simulink model "Assembly"  (R2022b)
settings: Solver=FixedStepAuto  StartTime=0.0  StopTime=20  FixedStep=0.001  RelTol=1e-3
model workspace: external: MATLAB File D:\Bw Jiang\Documents\FCS\DuctedFanUAV\Assembly_DataFile.m (data not in the file)
undefined symbols (not defined in the file or in its folder): DiscIntNeverNeededParam, smiData, X, Y, Z
libraries: sm_lib x26, nesl_utility x21, slpidlib x18, simulink_extras x5, simulink x4, shared6dof x2
(part 1 of 4)
settings Model: PacingRate=0.250000  Creator=Bw Jiang  LastModifiedBy=Bw Jiang
settings DebuggingCC: UnconnectedInputMsg=warning  UnconnectedOutputMsg=warning  UnconnectedLineMsg=warning
settings ModelReferenceCC: EnableRefExpFcnMdlSchedulingChecks=on
settings RTWCC: DLArmComputeVersion=19.05

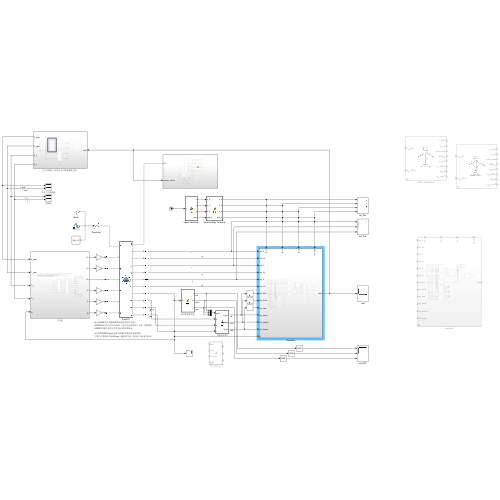
[thumbnail: Simulink's stored preview of the top-level diagram]
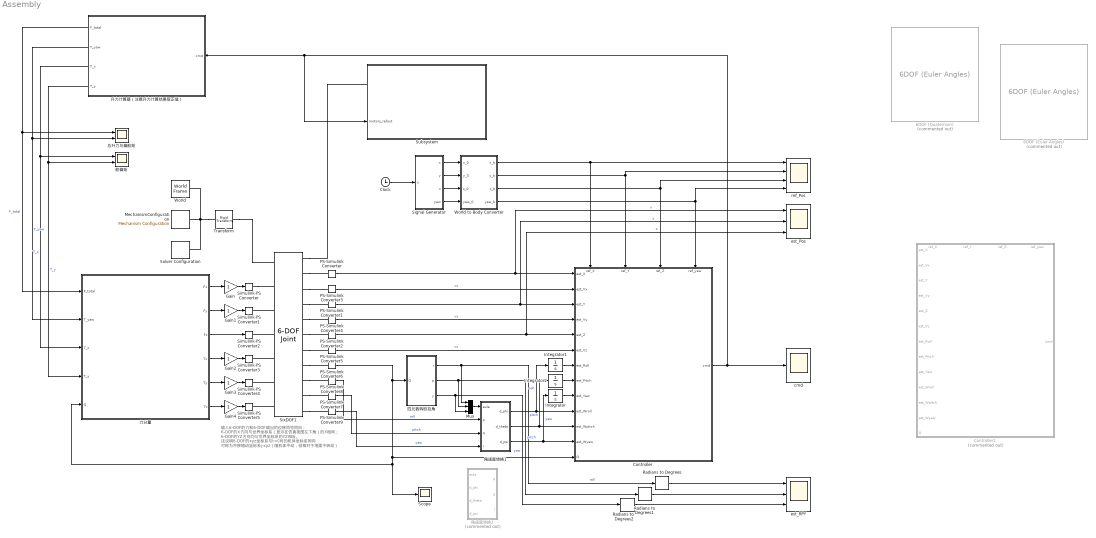
== system Assembly ==
  note: 输入6-DOF的力和6-DOF输出的位移同号同向；
      | 6-DOF的X方向与世界坐标系（显示在仿真视图左下角）的X相同；
      | 6-DOF的YZ方向均与世界坐标系的YZ相反。
      |
      | 这说明6-DOF的xyz坐标系与t=0时的机体坐标系同向
      | 可称为平移随动坐标系j-xyz（随机体平动，但相对于地面不转动）
  6DOF (Euler Angles) : shared6dof/6DOF (Euler Angles)  Commented=on  units=Metric (MKS)  mtype=Fixed  rep=Euler Angles  xme_0=[0 0 0]  Vm_0=[0 0 0]  eul_0=[0 0 0]  pm_0=[0 0 0]  mass_0=1.0  mass_e=0.5  mass_f=2.0  inertia=eye(3)  inertia_e=eye(3)  inertia_f=2*eye(3)  k_quat=1.0  vre_flag=on  abi_flag=off  aMode=0  xme_statename=''  Vm_statename=''  eul_statename=''  quat_statename=''  pm_statename=''  mass_statename=''
  6DOF (Quaternion) : shared6dof/6DOF (Euler Angles)  Commented=on  units=Metric (MKS)  mtype=Fixed  rep=Quaternion  xme_0=[0 0 0]  Vm_0=[0 0 0]  eul_0=[0 0 0]  pm_0=[0 0 0]  mass_0=1.0  mass_e=0.5  mass_f=2.0  inertia=eye(3)  inertia_e=eye(3)  inertia_f=2*eye(3)  k_quat=1.0  vre_flag=on  abi_flag=off  aMode=0  xme_statename=''  Vm_statename=''  eul_statename=''  quat_statename=''  pm_statename=''  mass_statename=''
  Clock : Clock
  Controller : Subsystem
      settings: PortSchema="{\"entries\":[{\"content\":{\"sides\":[{\"content\":{\"connectorIds\":[\"In1\",\"In2\",\"In3\",\"In4\",\"In5\",\"In6\",\"In7\",\"In8\",\"In9\",\"In10\",\"In11\",\"In12\",\"In13\"]},\"type\":\"ConnectorPlacement.EquallySpacedRectSide\",\"uuid\":\"809a58d1-8f24-4346-a9a1-bdf3f40071a9\"},{\"content\":{\"connectorIds\":[\"Out1\"],\"side\":\"RIGHT\"},\"type\":\"ConnectorPlacement.EquallySpacedRectSide\",\"uuid\":\"e36db7a5-8644-49ff-9b48-8e381d81be19\"},{\"content\":{\"connectorIds\":[\"In14\",\"In15\",\"In16\",\"In17\"],\"side\":\"TOP\"},\"type\":\"ConnectorPlacement.EquallySpacedRectSide\",\"uuid\":\"d8c211b6-7652-4be5-9d63-16c6c31a5cb3\"}]},\"type\":\"ConnectorPlacement.EquallySpacedConnector\",\"uuid\":\"28a38415-8484-4982-8141-ea2d794bbc37\"}],\"packageUris\":[\"http://schema.mathworks.com/mf0/Connector/R2020b\"],\"version\":\"1.0\"}"
  Controller1 : Subsystem  Commented=on
      settings: PortSchema="{\"entries\":[{\"content\":{\"sides\":[{\"content\":{\"connectorIds\":[\"In1\",\"In2\",\"In3\",\"In4\",\"In5\",\"In6\",\"In7\",\"In8\",\"In9\",\"In10\",\"In11\",\"In12\",\"In13\"]},\"type\":\"ConnectorPlacement.EquallySpacedRectSide\",\"uuid\":\"809a58d1-8f24-4346-a9a1-bdf3f40071a9\"},{\"content\":{\"connectorIds\":[\"Out1\"],\"side\":\"RIGHT\"},\"type\":\"ConnectorPlacement.EquallySpacedRectSide\",\"uuid\":\"e36db7a5-8644-49ff-9b48-8e381d81be19\"},{\"content\":{\"connectorIds\":[\"In14\",\"In15\",\"In16\",\"In17\"],\"side\":\"TOP\"},\"type\":\"ConnectorPlacement.EquallySpacedRectSide\",\"uuid\":\"d8c211b6-7652-4be5-9d63-16c6c31a5cb3\"}]},\"type\":\"ConnectorPlacement.EquallySpacedConnector\",\"uuid\":\"28a38415-8484-4982-8141-ea2d794bbc37\"}],\"packageUris\":[\"http://schema.mathworks.com/mf0/Connector/R2020b\"],\"version\":\"1.0\"}"
  Gain{,1..4} (5 alike) : Gain
  Integrator : Integrator
  Integrator1 : Integrator
  Integrator2 : Integrator
  MechanismConfiguration : sm_lib/Utilities/Mechanism Configuration  UniformGravity=Constant  GravityVector=[0 0 -9.81]  GravityUnits=m/s^2  LinearizationDelta=0.001  JointModeTransitionNonlinearIterations=2
  Mux : Mux  Inputs=3
  PS-Simulink Converter{,1..9} (10 alike) : nesl_utility/PS-Simulink Converter  PhysicalDomain=network_engine_domain  SubClassName=ps_output  LeftPortType=input  RightPortType=output  PseudoPeriodic=off  Frequencies=[]  VectorFormat=1-D array  Unit=inherit  AffineConversion=off
  Radians to Degrees : simulink_extras/Transformations/Radians to Degrees
  Radians to Degrees1 : simulink_extras/Transformations/Radians to Degrees
  Radians to Degrees2 : simulink_extras/Transformations/Radians to Degrees
  Scope : Scope
  Signal Generator : MATLAB Function  TreatAsAtomicUnit=on
  Simulink-PS Converter{,1..5} (6 alike) : nesl_utility/Simulink-PS Converter  PhysicalDomain=network_engine_domain  SubClassName=ps_input  LeftPortType=input  RightPortType=output  PseudoPeriodic=off  Frequencies=[]  NoiseDistribution=none  NoiseParameters=[]  Unit=1  AffineConversion=off  FilteringAndDerivatives=provide  SimscapeFilterOrder=1  InputFilterTimeConstant=0.001  UdotUserProvided=0
  SixDOF1 : sm_lib/Joints/6-DOF Joint  JointMode=Normal  SenseConstraintForce=off  SenseConstraintForceX=off  SenseConstraintForceY=off  SenseConstraintForceZ=off  SenseConstraintTorque=off  SenseConstraintTorqueX=off  SenseConstraintTorqueY=off  SenseConstraintTorqueZ=off  SenseTotalForce=off  SenseTotalForceX=off  SenseTotalForceY=off  SenseTotalForceZ=off  SenseTotalTorque=off  SenseTotalTorqueX=off  SenseTotalTorqueY=off  SenseTotalTorqueZ=off  CompositeWrenchDir=FollowerOnBase  CompositeWrenchFrame=BaseFrame  PxEquilibriumPosition=0  PxEquilibriumPositionUnits=m  PxSpringStiffness=0  PxSpringStiffnessUnits=N/m  PxDampingCoefficient=0  PxDampingCoefficientUnits=N/(m/s)  PxTorqueActuationMode=InputTorque  PxMotionActuationMode=ComputedMotion  PxSensePosition=on  PxSenseVelocity=on  PxSenseAcceleration=off  PxSenseTorqueForce=off  PxSenseLowerLimitTorqueForce=off  PxSenseUpperLimitTorqueForce=off  PxLowerLimitSpecify=off  PxLowerLimitBound=-1  PxLowerLimitBoundUnits=m  PxLowerLimitStiffness=1e6  PxLowerLimitStiffnessUnits=N/m  PxLowerLimitDamping=1e3  PxLowerLimitDampingUnits=N/(m/s)  PxLowerLimitTransitionRegionWidth=1e-4  PxLowerLimitTransitionRegionWidthUnits=m  PxUpperLimitSpecify=off  PxUpperLimitBound=1  PxUpperLimitBoundUnits=m  PxUpperLimitStiffness=1e6  PxUpperLimitStiffnessUnits=N/m  PxUpperLimitDamping=1e3  PxUpperLimitDampingUnits=N/(m/s)  PxUpperLimitTransitionRegionWidth=1e-4  PxUpperLimitTransitionRegionWidthUnits=m  PxPositionTargetSpecify=off  PxPositionTargetPriority=High  PxPositionTargetValue=0  PxPositionTargetValueUnits=m  PxVelocityTargetSpecify=off  PxVelocityTargetPriority=High  PxVelocityTargetValue=0  PxVelocityTargetValueUnits=m/s  PyEquilibriumPosition=0  PyEquilibriumPositionUnits=m  PySpringStiffness=0  PySpringStiffnessUnits=N/m  PyDampingCoefficient=0  PyDampingCoefficientUnits=N/(m/s)  PyTorqueActuationMode=InputTorque  PyMotionActuationMode=ComputedMotion  PySensePosition=on  PySenseVelocity=on  PySenseAcceleration=off  PySenseTorqueForce=off  PySenseLowerLimitTorqueForce=off  PySenseUpperLimitTorqueForce=off  PyLowerLimitSpecify=off  PyLowerLimitBound=-1  PyLowerLimitBoundUnits=m  PyLowerLimitStiffness=1e6  PyLowerLimitStiffnessUnits=N/m  PyLowerLimitDamping=1e3  PyLowerLimitDampingUnits=N/(m/s)  PyLowerLimitTransitionRegionWidth=1e-4  PyLowerLimitTransitionRegionWidthUnits=m  PyUpperLimitSpecify=off  PyUpperLimitBound=1  PyUpperLimitBoundUnits=m  PyUpperLimitStiffness=1e6  PyUpperLimitStiffnessUnits=N/m  PyUpperLimitDamping=1e3  PyUpperLimitDampingUnits=N/(m/s)  PyUpperLimitTransitionRegionWidth=1e-4  PyUpperLimitTransitionRegionWidthUnits=m  PyPositionTargetSpecify=off  PyPositionTargetPriority=High  PyPositionTargetValue=0  PyPositionTargetValueUnits=m  PyVelocityTargetSpecify=off  PyVelocityTargetPriority=High  PyVelocityTargetValue=0  PyVelocityTargetValueUnits=m/s  PzEquilibriumPosition=0  PzEquilibriumPositionUnits=m  PzSpringStiffness=0  PzSpringStiffnessUnits=N/m  PzDampingCoefficient=0  PzDampingCoefficientUnits=N/(m/s)  PzTorqueActuationMode=InputTorque  PzMotionActuationMode=ComputedMotion  PzSensePosition=on  PzSenseVelocity=on  PzSenseAcceleration=off  PzSenseTorqueForce=off  PzSenseLowerLimitTorqueForce=off  PzSenseUpperLimitTorqueForce=off  PzLowerLimitSpecify=off  PzLowerLimitBound=-1  PzLowerLimitBoundUnits=m  PzLowerLimitStiffness=1e6  PzLowerLimitStiffnessUnits=N/m  PzLowerLimitDamping=1e3  PzLowerLimitDampingUnits=N/(m/s)  PzLowerLimitTransitionRegionWidth=1e-4  PzLowerLimitTransitionRegionWidthUnits=m  PzUpperLimitSpecify=off  PzUpperLimitBound=1  PzUpperLimitBoundUnits=m  PzUpperLimitStiffness=1e6  PzUpperLimitStiffnessUnits=N/m  PzUpperLimitDamping=1e3  PzUpperLimitDampingUnits=N/(m/s)  PzUpperLimitTransitionRegionWidth=1e-4  PzUpperLimitTransitionRegionWidthUnits=m  PzPositionTargetSpecify=off  PzPositionTargetPriority=High  PzPositionTargetValue=0  PzPositionTargetValueUnits=m  PzVelocityTargetSpecify=off  PzVelocityTargetPriority=High  PzVelocityTargetValue=0  PzVelocityTargetValueUnits=m/s  SphEqPosRotationMethod=None  SphEqPosRotationAngleUnits=deg  SphEqPosRotationStandardAxis=+Z  SphEqPosRotationAngle=0.0  SphEqPosRotationArbitraryAxis=[0 0 1]  SphEqPosFollAlignAxisA=+X  SphEqPosBaseAlignAxisA=+Y  SphEqPosFollAlignAxisB=+Y  SphEqPosBaseAlignAxisB=+Z  SphEqPosRotationSequenceAxes=FollowerAxes  SphEqPosRotationSequence=XYX  SphEqPosRotationSequenceAngles=[0 0 0]  SphEqPosRotationSequenceAnglesUnits=deg  SphEqPosRotationMatrix=[1 0 0; 0 1 0; 0 0 1]  SphEqPosQuaternion=[1 0 0 0]  SphSpringStiffness=0  SphSpringStiffnessUnits=N*m/deg  SphDampingCoefficient=0  SphDampingCoefficientUnits=N*m/(deg/s)  SphActuateTorqueX=on  SphActuateTorqueY=on  SphActuateTorqueZ=on  SphActuateTorque=off  SphTorqueActuationMode=InputTorque  SphMotionActuationMode=ComputedMotion  SphActuationFrame=BaseFrame  SphSensePosition=on  SphSenseVelocityX=on  SphSenseVelocityY=on  SphSenseVelocityZ=on  SphSenseVelocity=off  SphSenseAccelerationX=off  SphSenseAccelerationY=off  SphSenseAccelerationZ=off  SphSenseAcceleration=off  SphSenseTorqueX=off  SphSenseTorqueY=off  SphSenseTorqueZ=off  SphSenseTorqueForce=off  SphSenseLowerLimitTorqueMag=off  SphSenseUpperLimitTorqueMag=off  SphSensingFrame=FollowerFrame  SphLowerLimitSpecify=off  SphLowerLimitBound=15  SphLowerLimitBoundUnits=deg  SphLowerLimitStiffness=1e4  SphLowerLimitStiffnessUnits=N*m/deg  SphLowerLimitDamping=10  SphLowerLimitDampingUnits=N*m/(deg/s)  SphLowerLimitTransitionRegionWidth=0.1  SphLowerLimitTransitionRegionWidthUnits=deg  SphUpperLimitSpecify=off  SphUpperLimitBound=45  SphUpperLimitBoundUnits=deg  SphUpperLimitStiffness=1e4  SphUpperLimitStiffnessUnits=N*m/deg  SphUpperLimitDamping=10  SphUpperLimitDampingUnits=N*m/(deg/s)  SphUpperLimitTransitionRegionWidth=0.1  SphUpperLimitTransitionRegionWidthUnits=deg  SphPositionTargetRotationMethod=None  SphPositionTargetRotationAngleUnits=deg  SphPositionTargetRotationStandardAxis=+Z  SphPositionTargetRotationAngle=0.0  SphPositionTargetRotationArbitraryAxis=[0 0 1]  SphPositionTargetFollAlignAxisA=+X  SphPositionTargetBaseAlignAxisA=+Y  SphPositionTargetFollAlignAxisB=+Y  SphPositionTargetBaseAlignAxisB=+Z  SphPositionTargetRotationSequenceAxes=FollowerAxes  SphPositionTargetRotationSequence=XYX  SphPositionTargetRotationSequenceAngles=[0 0 0]  SphPositionTargetRotationSequenceAnglesUnits=deg  SphPositionTargetRotationMatrix=[1 0 0; 0 1 0; 0 0 1]  SphPositionTargetQuaternion=[1 0 0 0]  SphPositionTargetSpecify=off  SphPositionTargetPriority=High  SphVelocityTargetValue=[0 0 0]  SphVelocityTargetValueUnits=deg/s  SphVelocityTargetSpecify=off  SphVelocityTargetPriority=High  SphVelocityTargetInFollowerFrame=on
  Solver Configuration : nesl_utility/Solver Configuration  PhysicalDomain=network_engine_domain  SubClassName=solver  LeftPortType=input  RightPortType=generic  Tones=[]  Harmonics=[]  SimulateNoise=off  Profile=off  UseLocalSampling=off  EnableSwitchedLinearOptims=on  FrequencyDomain=off  UseCCode=off  RelTol=0.001  AbsTol=1e-06  MinStep=1e-09  ToWorkspace=off  RevertToSquareIcSolve=off  NumHomotopyIterations=100  PhasorMode=off  PhasorModeNumHarmonics=1  ConsistencySolver=NEWTON_FTOL  IndexReductionMethod=DerivativeReplacement  DoDC=off  ResidualTolerance=1e-09  ConsistencyTolSource=GLOBAL  ConsistencyAbsTol=0.001  ConsistencyRelTol=0.001  ConsistencyTolFactor=0.001  UseLocalSolver=off  LocalSolverChoice=NE_BACKWARD_EULER_ADVANCER  ResolveIndetEquations=on  FunctionEvalNumThread=1  LocalSolverSampleTime=0.001  DoFixedCost=off  MaxNonlinIter=3  MaxModeIter=2  ComputeImpulses=off  ImpulseIterations=2  LinearAlgebra=auto  LinearAlgebraNumThread=0  EquationFormulation=NE_TIME_EF  DelaysMemoryBudget=1024  AutomaticFiltering=on  FilteringTimeConstant=0.001  PartitionStorageMethod=AS_NEEDED  PartitionMemoryBudget=1024  PartitionMethod=ROBUST
  Subsystem : Subsystem
      settings: PortSchema="{\"entries\":[{\"content\":{\"sides\":[{\"content\":{\"connectorIds\":[\"LConn1\",\"In1\"]},\"type\":\"ConnectorPlacement.EquallySpacedRectSide\",\"uuid\":\"bb094976-7db4-48e7-8e36-7ac433ff8066\"},{\"content\":{\"connectorIds\":[],\"side\":\"RIGHT\"},\"type\":\"ConnectorPlacement.EquallySpacedRectSide\",\"uuid\":\"dd79df54-9b88-42e2-b922-2d03729e012c\"},{\"content\":{\"connectorIds\":[],\"side\":\"TOP\"},\"type\":\"ConnectorPlacement.EquallySpacedRectSide\",\"uuid\":\"8c3b65bd-df1f-4b29-9de8-9f0a1a13e75c\"}]},\"type\":\"ConnectorPlacement.EquallySpacedConnector\",\"uuid\":\"8aa4c324-e909-40a5-a887-f09e9aac14b3\"}],\"packageUris\":[\"http://schema.mathworks.com/mf0/Connector/R2020b\"],\"version\":\"1.0\"}"
  Transform : sm_lib/Frames and Transforms/Rigid Transform  TranslationMethod=Cartesian  TranslationStandardOffset=0  TranslationLengthUnit=mm  TranslationStandardAxis=+Z  TranslationCartesianOffset=smiData.RigidTransform(9).translation  TranslationROffset=0  TranslationROffsetUnits=m  TranslationZOffset=0  TranslationZOffsetUnits=m  TranslationThetaOffset=0  TranslationThetaOffsetUnits=deg  RotationMethod=RotationSequence  RotationAngleUnits=rad  RotationStandardAxis=+Z  RotationAngle=smiData.RigidTransform(9).angle  RotationArbitraryAxis=smiData.RigidTransform(9).axis  FollAlignAxisA=+X  BaseAlignAxisA=+Y  FollAlignAxisB=+Y  BaseAlignAxisB=+Z  RotationSequenceAxes=FollowerAxes  RotationSequence=XYX  RotationSequenceAngles=[180 0 0]  RotationSequenceAnglesUnits=deg  RotationMatrix=[1 0 0; 0 1 0; 0 0 1]  Quaternion=[1 0 0 0]
  World : sm_lib/Frames and Transforms/World Frame
  World to Body Converter : MATLAB Function  TreatAsAtomicUnit=on
  cmd : Scope
  est_Pos : Scope  NumInputPorts=3
  est_RPY : Scope  NumInputPorts=3
  ref_Pos : Scope  NumInputPorts=4
  力分量 : Subsystem
  升力计算器（注意升力计算结果取正值） : Subsystem
      settings: PortSchema="{\"entries\":[{\"content\":{\"sides\":[{\"content\":{\"connectorIds\":[\"Out1\",\"Out2\",\"Out3\",\"Out4\"]},\"type\":\"ConnectorPlacement.EquallySpacedRectSide\",\"uuid\":\"21ecbfb4-a858-465b-a1bc-21a9ca7a9f3e\"},{\"content\":{\"connectorIds\":[\"In1\"],\"side\":\"RIGHT\"},\"type\":\"ConnectorPlacement.EquallySpacedRectSide\",\"uuid\":\"c558c55c-c027-40b6-93c1-e1a586e493e8\"},{\"content\":{\"connectorIds\":[],\"side\":\"TOP\"},\"type\":\"ConnectorPlacement.EquallySpacedRectSide\",\"uuid\":\"3cee70e1-31e7-4918-8bab-ddb1926e8bf9\"}]},\"type\":\"ConnectorPlacement.EquallySpacedConnector\",\"uuid\":\"ca7cf621-4077-4d76-982c-1b5c8640684e\"}],\"packageUris\":[\"http://schema.mathworks.com/mf0/Connector/R2020b\"],\"version\":\"1.0\"}"
  四元数转欧拉角 : MATLAB Function  TreatAsAtomicUnit=on
  总升力与偏航矩 : Scope  NumInputPorts=2
  舵偏矩 : Scope  NumInputPorts=2
  角速度转换1 : MATLAB Function  TreatAsAtomicUnit=on
  角速度转换2 : MATLAB Function  Commented=on  TreatAsAtomicUnit=on
  wires:
  四元数转欧拉角/2(p) -> Radians to Degrees1/1, Mux/2  "pitch"
  PS-Simulink Converter8/1 -> 角速度转换1/2(p)  "roll"
  升力计算器（注意升力计算结果取正值）/3(T_x) -> 舵偏矩/1, 力分量/3(T_x)  "T_x"
  升力计算器（注意升力计算结果取正值）/2(T_yaw) -> 总升力与偏航矩/2, 力分量/2(T_yaw)  "T_yaw"
  Controller/1(cmd) -> Subsystem/1(motors_refout), 升力计算器（注意升力计算结果取正值）/1(cmd), cmd/1
  World to Body Converter/4(yaw_b) -> ref_Pos/4, Controller/17(ref_yaw)
  World to Body Converter/1(x_b) -> ref_Pos/1, Controller/14(ref_X)
  PS-Simulink Converter/1 -> est_Pos/1, Controller/1(est_X)  "x"
  升力计算器（注意升力计算结果取正值）/1(F_total) -> 力分量/1(F_total), 总升力与偏航矩/1  "F_total"
  四元数转欧拉角/1(r) -> Radians to Degrees/1, Mux/1  "roll"
  World to Body Converter/2(y_b) -> ref_Pos/2, Controller/15(ref_Y)
  PS-Simulink Converter2/1 -> est_Pos/3, Controller/5(est_Z)  "z"
  PS-Simulink Converter1/1 -> est_Pos/2, Controller/3(est_Y)  "y"
  PS-Simulink Converter6/1 -> Scope/1, 力分量/5(Q), Controller/13(Q), 四元数转欧拉角/1(Q)
  PS-Simulink Converter7/1 -> 角速度转换1/3(q)  "pitch"
  PS-Simulink Converter9/1 -> 角速度转换1/4(r)  "yaw"
  PS-Simulink Converter3/1 -> Controller/2(est_Vx)  "vx"
  四元数转欧拉角/3(y) -> Radians to Degrees2/1, Mux/3  "yaw"
  升力计算器（注意升力计算结果取正值）/4(T_y) -> 舵偏矩/2, 力分量/4(T_y)  "T_y"
  PS-Simulink Converter5/1 -> Controller/6(est_Vz)  "vz"
  PS-Simulink Converter4/1 -> Controller/4(est_Vy)  "vy"
  World to Body Converter/3(z_b) -> ref_Pos/3, Controller/16(ref_Z)
  力分量/2(Fy) -> Gain1/1
  力分量/3(Fz) -> Simulink-PS Converter2/1
  力分量/4(Tx) -> Gain2/1
  力分量/5(Ty) -> Gain3/1
  力分量/6(Tz) -> Gain4/1
  力分量/1(Fx) -> Gain/1
  Signal Generator/4(yaw) -> World to Body Converter/4(yaw_0)
  Signal Generator/3(z) -> World to Body Converter/3(z_0)
  Signal Generator/1(x) -> World to Body Converter/1(x_0)
  Clock/1 -> Signal Generator/1(u)
  Signal Generator/2(y) -> World to Body Converter/2(y_0)
  Radians to Degrees/1 -> est_RPY/1
  Radians to Degrees1/1 -> est_RPY/2
  Radians to Degrees2/1 -> est_RPY/3
  Gain/1 -> Simulink-PS Converter/1
  Gain1/1 -> Simulink-PS Converter1/1
  Gain2/1 -> Simulink-PS Converter3/1
  Gain3/1 -> Simulink-PS Converter4/1
  Gain4/1 -> Simulink-PS Converter5/1
  Mux/1 -> 角速度转换1/1(eula)
  角速度转换1/1(d_phi) -> Integrator1/1, Controller/10(est_Wroll)  "roll"
  角速度转换1/2(d_theta) -> Integrator2/1, Controller/11(est_Wpitch)  "pitch"
  角速度转换1/3(d_psi) -> Integrator/1, Controller/12(est_Wyaw)  "yaw"
  Integrator/1 -> Controller/9(est_Yaw)
  Integrator1/1 -> Controller/7(est_Roll)
  Integrator2/1 -> Controller/8(est_Pitch)
  connections:
  Transform/LConn1 -- MechanismConfiguration/RConn1 -- Solver Configuration/RConn1 -- World/RConn1
  SixDOF1/RConn11 -- PS-Simulink Converter9/LConn1
  SixDOF1/LConn3 -- Simulink-PS Converter1/RConn1
  SixDOF1/RConn1 -- Subsystem/LConn1
  SixDOF1/RConn3 -- PS-Simulink Converter3/LConn1
  SixDOF1/LConn6 -- Simulink-PS Converter4/RConn1
  Simulink-PS Converter/RConn1 -- SixDOF1/LConn2
  SixDOF1/RConn2 -- PS-Simulink Converter/LConn1
  SixDOF1/RConn10 -- PS-Simulink Converter7/LConn1
  SixDOF1/RConn8 -- PS-Simulink Converter6/LConn1
  SixDOF1/LConn4 -- Simulink-PS Converter2/RConn1
  SixDOF1/RConn5 -- PS-Simulink Converter4/LConn1
  SixDOF1/LConn5 -- Simulink-PS Converter3/RConn1
  SixDOF1/LConn7 -- Simulink-PS Converter5/RConn1
  SixDOF1/RConn7 -- PS-Simulink Converter5/LConn1
  SixDOF1/RConn4 -- PS-Simulink Converter1/LConn1
  SixDOF1/RConn9 -- PS-Simulink Converter8/LConn1
  SixDOF1/RConn6 -- PS-Simulink Converter2/LConn1
  Transform/RConn1 -- SixDOF1/LConn1

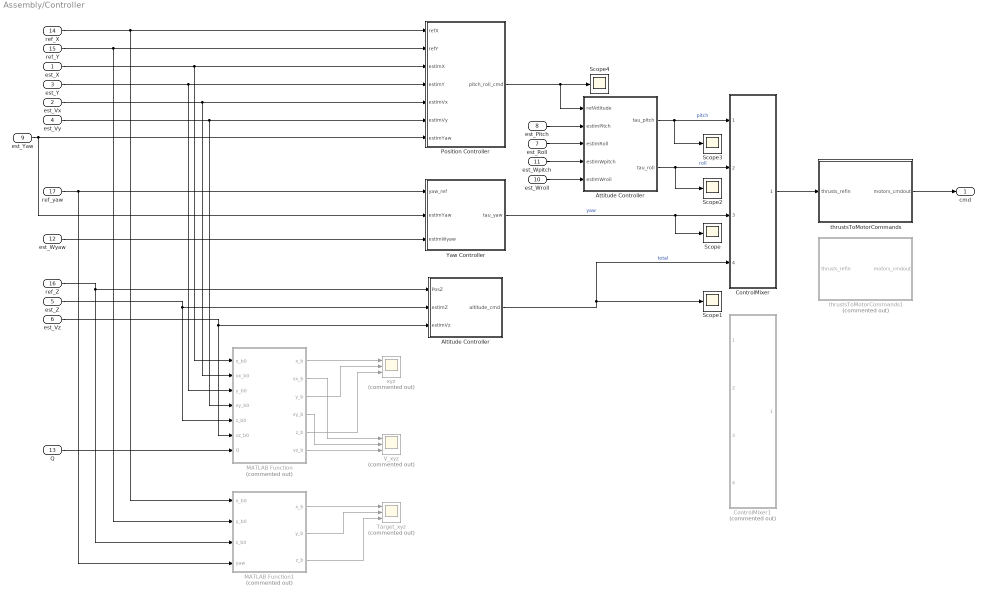
== system Assembly/Controller ==
  est_X : Inport
  est_Vx : Inport  Port=2
  est_Y : Inport  Port=3
  est_Vy : Inport  Port=4
  est_Z : Inport  Port=5
  est_Vz : Inport  Port=6
  est_Roll : Inport  Port=7
  est_Pitch : Inport  Port=8
  est_Yaw : Inport  Port=9
  est_Wroll : Inport  Port=10
  est_Wpitch : Inport  Port=11
  est_Wyaw : Inport  Port=12
  Q : Inport  Port=13
  ref_X : Inport  Port=14
  ref_Y : Inport  Port=15
  ref_Z : Inport  Port=16
  ref_yaw : Inport  Port=17
  Altitude Controller : Subsystem
  Attitude Controller : Subsystem
  ControlMixer : Subsystem
  ControlMixer1 : Subsystem  Commented=on
  MATLAB Function : MATLAB Function  Commented=on  TreatAsAtomicUnit=on
  MATLAB Function1 : MATLAB Function  Commented=on  TreatAsAtomicUnit=on
  Position Controller : Subsystem
  Scope{,1..4} (5 alike) : Scope
  Target_xyz : Scope  Commented=on  NumInputPorts=3
  V_xyz : Scope  Commented=on  NumInputPorts=3
  Yaw Controller : Subsystem
  thrustsToMotorCommands : Subsystem
  thrustsToMotorCommands1 : Subsystem  Commented=on
  xyz : Scope  Commented=on  NumInputPorts=3
  cmd : Outport  VectorParamsAs1DForOutWhenUnconnected=off
  wires:
  ControlMixer/1(thrusts_refout) -> thrustsToMotorCommands/1(thrusts_refin)
  est_X/1 -> MATLAB Function/1(x_b0), Position Controller/3(estimX)
  est_Pitch/1 -> Attitude Controller/2(estimPitch)
  est_Vz/1 -> MATLAB Function/6(vz_b0), Altitude Controller/3(estimVz)
  ref_X/1 -> MATLAB Function1/1(x_b0), Position Controller/1(refX)
  est_Z/1 -> MATLAB Function/5(z_b0), Altitude Controller/2(estimZ)
  Attitude Controller/1(tau_pitch) -> ControlMixer/1(tau_pitch), Scope3/1  "pitch"
  ref_yaw/1 -> MATLAB Function1/4(yaw), Yaw Controller/1(yaw_ref)
  est_Y/1 -> MATLAB Function/3(y_b0), Position Controller/4(estimY)
  ref_Z/1 -> MATLAB Function1/3(z_b0), Altitude Controller/1(PosZ)
  Position Controller/1(pitch_roll_cmd) -> Scope4/1, Attitude Controller/1(refAttitude)
  est_Wroll/1 -> Attitude Controller/5(estimWroll)
  ref_Y/1 -> MATLAB Function1/2(y_b0), Position Controller/2(refY)
  Attitude Controller/2(tau_roll) -> ControlMixer/2(tau_roll), Scope2/1  "roll"
  est_Vx/1 -> MATLAB Function/2(vx_b0), Position Controller/5(estimVx)
  est_Wyaw/1 -> Yaw Controller/3(estimWyaw)
  Altitude Controller/1(altitude_cmd) -> ControlMixer/4(totalThrust), Scope1/1  "total"
  est_Yaw/1 -> Position Controller/7(estimYaw), Yaw Controller/2(estimYaw)
  est_Wpitch/1 -> Attitude Controller/4(estimWpitch)
  Yaw Controller/1(tau_yaw) -> ControlMixer/3(tau_yaw), Scope/1  "yaw"
  est_Vy/1 -> MATLAB Function/4(vy_b0), Position Controller/6(estimVy)
  thrustsToMotorCommands/1(motors_cmdout) -> cmd/1
  est_Roll/1 -> Attitude Controller/3(estimRoll)
  Q/1 -> MATLAB Function/7(Q)
  MATLAB Function/1(x_b) -> xyz/1
  MATLAB Function/3(y_b) -> xyz/2
  MATLAB Function/5(z_b) -> xyz/3
  MATLAB Function/2(vx_b) -> V_xyz/1
  MATLAB Function/4(vy_b) -> V_xyz/2
  MATLAB Function/6(vz_b) -> V_xyz/3
  MATLAB Function1/1(x_b) -> Target_xyz/1
  MATLAB Function1/2(y_b) -> Target_xyz/2
  MATLAB Function1/3(z_b) -> Target_xyz/3

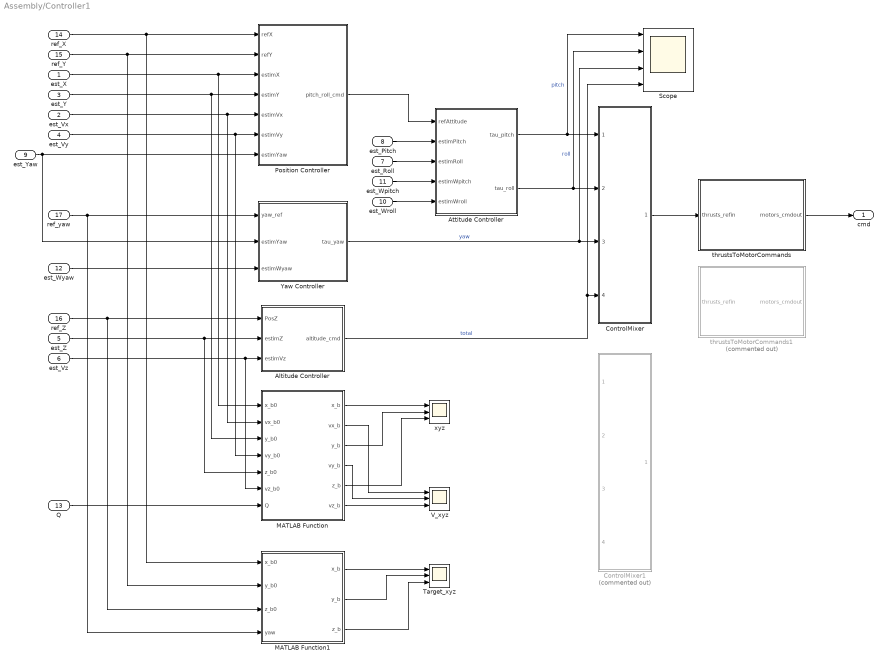
== system Assembly/Controller1 ==
  est_X : Inport
  est_Vx : Inport  Port=2
  est_Y : Inport  Port=3
  est_Vy : Inport  Port=4
  est_Z : Inport  Port=5
  est_Vz : Inport  Port=6
  est_Roll : Inport  Port=7
  est_Pitch : Inport  Port=8
  est_Yaw : Inport  Port=9
  est_Wroll : Inport  Port=10
  est_Wpitch : Inport  Port=11
  est_Wyaw : Inport  Port=12
  Q : Inport  Port=13
  ref_X : Inport  Port=14
  ref_Y : Inport  Port=15
  ref_Z : Inport  Port=16
  ref_yaw : Inport  Port=17
  Altitude Controller : Subsystem
  Attitude Controller : Subsystem
  ControlMixer : Subsystem
  ControlMixer1 : Subsystem  Commented=on
  MATLAB Function : MATLAB Function  TreatAsAtomicUnit=on
  MATLAB Function1 : MATLAB Function  TreatAsAtomicUnit=on
  Position Controller : Subsystem
  Scope : Scope  NumInputPorts=4
  Target_xyz : Scope  NumInputPorts=3
  V_xyz : Scope  NumInputPorts=3
  Yaw Controller : Subsystem
  thrustsToMotorCommands : Subsystem
  thrustsToMotorCommands1 : Subsystem  Commented=on
  xyz : Scope  NumInputPorts=3
  cmd : Outport  VectorParamsAs1DForOutWhenUnconnected=off
  wires:
  ControlMixer/1(thrusts_refout) -> thrustsToMotorCommands/1(thrusts_refin)
  est_X/1 -> MATLAB Function/1(x_b0), Position Controller/3(estimX)
  est_Pitch/1 -> Attitude Controller/2(estimPitch)
  est_Vz/1 -> MATLAB Function/6(vz_b0), Altitude Controller/3(estimVz)
  ref_X/1 -> MATLAB Function1/1(x_b0), Position Controller/1(refX)
  est_Z/1 -> MATLAB Function/5(z_b0), Altitude Controller/2(estimZ)
  Attitude Controller/1(tau_pitch) -> ControlMixer/1(tau_pitch), Scope/1  "pitch"
  ref_yaw/1 -> MATLAB Function1/4(yaw), Yaw Controller/1(yaw_ref)
  est_Y/1 -> MATLAB Function/3(y_b0), Position Controller/4(estimY)
  ref_Z/1 -> MATLAB Function1/3(z_b0), Altitude Controller/1(PosZ)
  Position Controller/1(pitch_roll_cmd) -> Attitude Controller/1(refAttitude)
  est_Wroll/1 -> Attitude Controller/5(estimWroll)
  ref_Y/1 -> MATLAB Function1/2(y_b0), Position Controller/2(refY)
  Attitude Controller/2(tau_roll) -> ControlMixer/2(tau_roll), Scope/2  "roll"
  est_Vx/1 -> MATLAB Function/2(vx_b0), Position Controller/5(estimVx)
  est_Wyaw/1 -> Yaw Controller/3(estimWyaw)
  Altitude Controller/1(altitude_cmd) -> Scope/4, ControlMixer/4(totalThrust)  "total"
  est_Yaw/1 -> Position Controller/7(estimYaw), Yaw Controller/2(estimYaw)
  est_Wpitch/1 -> Attitude Controller/4(estimWpitch)
  Yaw Controller/1(tau_yaw) -> ControlMixer/3(tau_yaw), Scope/3  "yaw"
  est_Vy/1 -> MATLAB Function/4(vy_b0), Position Controller/6(estimVy)
  thrustsToMotorCommands/1(motors_cmdout) -> cmd/1
  est_Roll/1 -> Attitude Controller/3(estimRoll)
  Q/1 -> MATLAB Function/7(Q)
  MATLAB Function/1(x_b) -> xyz/1
  MATLAB Function/3(y_b) -> xyz/2
  MATLAB Function/5(z_b) -> xyz/3
  MATLAB Function/2(vx_b) -> V_xyz/1
  MATLAB Function/4(vy_b) -> V_xyz/2
  MATLAB Function/6(vz_b) -> V_xyz/3
  MATLAB Function1/1(x_b) -> Target_xyz/1
  MATLAB Function1/2(y_b) -> Target_xyz/2
  MATLAB Function1/3(z_b) -> Target_xyz/3

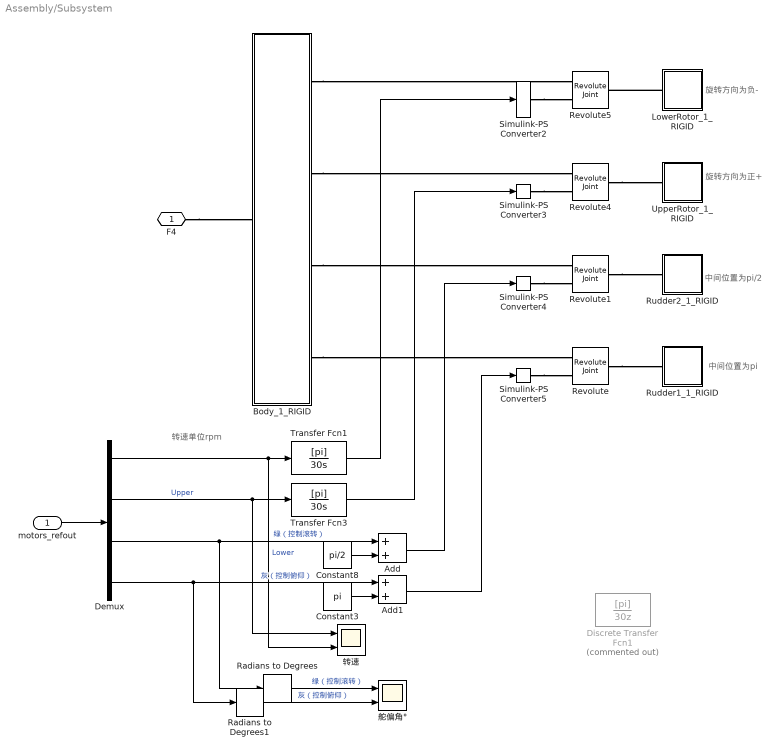
== system Assembly/Subsystem ==
  note: 转速单位rpm
  note: 旋转方向为正+
  note: 旋转方向为负-
  note: 中间位置为pi
  note: 中间位置为pi/2
  motors_refout : Inport
  Add : Sum
  Add1 : Sum
  Body_1_RIGID : Subsystem
  Constant3 : Constant  Value=pi
  Constant8 : Constant  Value=pi/2
  Demux : Demux
  Discrete Transfer Fcn1 : DiscreteTransferFcn  Commented=on  Numerator=[pi]  Denominator=[30 0]
  LowerRotor_1_RIGID : Subsystem
  Radians to Degrees : simulink_extras/Transformations/Radians to Degrees
  Radians to Degrees1 : simulink_extras/Transformations/Radians to Degrees
  Revolute : sm_lib/Joints/Revolute Joint  JointMode=Normal  SenseConstraintForce=off  SenseConstraintForceX=off  SenseConstraintForceY=off  SenseConstraintForceZ=off  SenseConstraintTorque=off  SenseConstraintTorqueX=off  SenseConstraintTorqueY=off  SenseConstraintTorqueZ=off  SenseTotalForce=off  SenseTotalForceX=off  SenseTotalForceY=off  SenseTotalForceZ=off  SenseTotalTorque=off  SenseTotalTorqueX=off  SenseTotalTorqueY=off  SenseTotalTorqueZ=off  CompositeWrenchDir=FollowerOnBase  CompositeWrenchFrame=BaseFrame  EquilibriumPosition=0  EquilibriumPositionUnits=deg  SpringStiffness=0  SpringStiffnessUnits=N*m/deg  DampingCoefficient=0  DampingCoefficientUnits=N*m/(deg/s)  TorqueActuationMode=ComputedTorque  MotionActuationMode=InputMotion  SensePosition=off  SenseVelocity=off  SenseAcceleration=off  SenseTorqueForce=off  SenseLowerLimitTorqueForce=off  SenseUpperLimitTorqueForce=off  LowerLimitSpecify=off  LowerLimitBound=-90  LowerLimitBoundUnits=deg  LowerLimitStiffness=1e4  LowerLimitStiffnessUnits=N*m/deg  LowerLimitDamping=10  LowerLimitDampingUnits=N*m/(deg/s)  LowerLimitTransitionRegionWidth=0.1  LowerLimitTransitionRegionWidthUnits=deg  UpperLimitSpecify=off  UpperLimitBound=90  UpperLimitBoundUnits=deg  UpperLimitStiffness=1e4  UpperLimitStiffnessUnits=N*m/deg  UpperLimitDamping=10  UpperLimitDampingUnits=N*m/(deg/s)  UpperLimitTransitionRegionWidth=0.1  UpperLimitTransitionRegionWidthUnits=deg  PositionTargetSpecify=on  PositionTargetPriority=Low  PositionTargetValue=smiData.RevoluteJoint(1).Rz.Pos  PositionTargetValueUnits=deg  VelocityTargetSpecify=off  VelocityTargetPriority=High  VelocityTargetValue=0  VelocityTargetValueUnits=deg/s
  Revolute1 : sm_lib/Joints/Revolute Joint  JointMode=Normal  SenseConstraintForce=off  SenseConstraintForceX=off  SenseConstraintForceY=off  SenseConstraintForceZ=off  SenseConstraintTorque=off  SenseConstraintTorqueX=off  SenseConstraintTorqueY=off  SenseConstraintTorqueZ=off  SenseTotalForce=off  SenseTotalForceX=off  SenseTotalForceY=off  SenseTotalForceZ=off  SenseTotalTorque=off  SenseTotalTorqueX=off  SenseTotalTorqueY=off  SenseTotalTorqueZ=off  CompositeWrenchDir=FollowerOnBase  CompositeWrenchFrame=BaseFrame  EquilibriumPosition=0  EquilibriumPositionUnits=deg  SpringStiffness=0  SpringStiffnessUnits=N*m/deg  DampingCoefficient=0  DampingCoefficientUnits=N*m/(deg/s)  TorqueActuationMode=ComputedTorque  MotionActuationMode=InputMotion  SensePosition=off  SenseVelocity=off  SenseAcceleration=off  SenseTorqueForce=off  SenseLowerLimitTorqueForce=off  SenseUpperLimitTorqueForce=off  LowerLimitSpecify=off  LowerLimitBound=-90  LowerLimitBoundUnits=deg  LowerLimitStiffness=1e4  LowerLimitStiffnessUnits=N*m/deg  LowerLimitDamping=10  LowerLimitDampingUnits=N*m/(deg/s)  LowerLimitTransitionRegionWidth=0.1  LowerLimitTransitionRegionWidthUnits=deg  UpperLimitSpecify=off  UpperLimitBound=90  UpperLimitBoundUnits=deg  UpperLimitStiffness=1e4  UpperLimitStiffnessUnits=N*m/deg  UpperLimitDamping=10  UpperLimitDampingUnits=N*m/(deg/s)  UpperLimitTransitionRegionWidth=0.1  UpperLimitTransitionRegionWidthUnits=deg  PositionTargetSpecify=on  PositionTargetPriority=Low  PositionTargetValue=smiData.RevoluteJoint(2).Rz.Pos  PositionTargetValueUnits=deg  VelocityTargetSpecify=off  VelocityTargetPriority=High  VelocityTargetValue=0  VelocityTargetValueUnits=deg/s
  Revolute4 : sm_lib/Joints/Revolute Joint  JointMode=Normal  SenseConstraintForce=off  SenseConstraintForceX=off  SenseConstraintForceY=off  SenseConstraintForceZ=off  SenseConstraintTorque=off  SenseConstraintTorqueX=off  SenseConstraintTorqueY=off  SenseConstraintTorqueZ=off  SenseTotalForce=off  SenseTotalForceX=off  SenseTotalForceY=off  SenseTotalForceZ=off  SenseTotalTorque=off  SenseTotalTorqueX=off  SenseTotalTorqueY=off  SenseTotalTorqueZ=off  CompositeWrenchDir=FollowerOnBase  CompositeWrenchFrame=BaseFrame  EquilibriumPosition=0  EquilibriumPositionUnits=deg  SpringStiffness=0  SpringStiffnessUnits=N*m/deg  DampingCoefficient=0  DampingCoefficientUnits=N*m/(deg/s)  TorqueActuationMode=ComputedTorque  MotionActuationMode=InputMotion  SensePosition=off  SenseVelocity=off  SenseAcceleration=off  SenseTorqueForce=off  SenseLowerLimitTorqueForce=off  SenseUpperLimitTorqueForce=off  LowerLimitSpecify=off  LowerLimitBound=-90  LowerLimitBoundUnits=deg  LowerLimitStiffness=1e4  LowerLimitStiffnessUnits=N*m/deg  LowerLimitDamping=10  LowerLimitDampingUnits=N*m/(deg/s)  LowerLimitTransitionRegionWidth=0.1  LowerLimitTransitionRegionWidthUnits=deg  UpperLimitSpecify=off  UpperLimitBound=90  UpperLimitBoundUnits=deg  UpperLimitStiffness=1e4  UpperLimitStiffnessUnits=N*m/deg  UpperLimitDamping=10  UpperLimitDampingUnits=N*m/(deg/s)  UpperLimitTransitionRegionWidth=0.1  UpperLimitTransitionRegionWidthUnits=deg  PositionTargetSpecify=on  PositionTargetPriority=Low  PositionTargetValue=smiData.RevoluteJoint(3).Rz.Pos  PositionTargetValueUnits=deg  VelocityTargetSpecify=off  VelocityTargetPriority=High  VelocityTargetValue=0  VelocityTargetValueUnits=deg/s
  Revolute5 : sm_lib/Joints/Revolute Joint  JointMode=Normal  SenseConstraintForce=off  SenseConstraintForceX=off  SenseConstraintForceY=off  SenseConstraintForceZ=off  SenseConstraintTorque=off  SenseConstraintTorqueX=off  SenseConstraintTorqueY=off  SenseConstraintTorqueZ=off  SenseTotalForce=off  SenseTotalForceX=off  SenseTotalForceY=off  SenseTotalForceZ=off  SenseTotalTorque=off  SenseTotalTorqueX=off  SenseTotalTorqueY=off  SenseTotalTorqueZ=off  CompositeWrenchDir=FollowerOnBase  CompositeWrenchFrame=BaseFrame  EquilibriumPosition=0  EquilibriumPositionUnits=deg  SpringStiffness=0  SpringStiffnessUnits=N*m/deg  DampingCoefficient=0  DampingCoefficientUnits=N*m/(deg/s)  TorqueActuationMode=ComputedTorque  MotionActuationMode=InputMotion  SensePosition=off  SenseVelocity=off  SenseAcceleration=off  SenseTorqueForce=off  SenseLowerLimitTorqueForce=off  SenseUpperLimitTorqueForce=off  LowerLimitSpecify=off  LowerLimitBound=-90  LowerLimitBoundUnits=deg  LowerLimitStiffness=1e4  LowerLimitStiffnessUnits=N*m/deg  LowerLimitDamping=10  LowerLimitDampingUnits=N*m/(deg/s)  LowerLimitTransitionRegionWidth=0.1  LowerLimitTransitionRegionWidthUnits=deg  UpperLimitSpecify=off  UpperLimitBound=90  UpperLimitBoundUnits=deg  UpperLimitStiffness=1e4  UpperLimitStiffnessUnits=N*m/deg  UpperLimitDamping=10  UpperLimitDampingUnits=N*m/(deg/s)  UpperLimitTransitionRegionWidth=0.1  UpperLimitTransitionRegionWidthUnits=deg  PositionTargetSpecify=on  PositionTargetPriority=Low  PositionTargetValue=smiData.RevoluteJoint(4).Rz.Pos  PositionTargetValueUnits=deg  VelocityTargetSpecify=off  VelocityTargetPriority=High  VelocityTargetValue=0  VelocityTargetValueUnits=deg/s
  Rudder1_1_RIGID : Subsystem
  Rudder2_1_RIGID : Subsystem
  Simulink-PS Converter{2..5} (4 alike) : nesl_utility/Simulink-PS Converter  PhysicalDomain=network_engine_domain  SubClassName=ps_input  LeftPortType=input  RightPortType=output  PseudoPeriodic=off  Frequencies=[]  NoiseDistribution=none  NoiseParameters=[]  Unit=1  AffineConversion=off  FilteringAndDerivatives=filter  SimscapeFilterOrder=2  InputFilterTimeConstant=0.001  UdotUserProvided=2
  Transfer Fcn1 : TransferFcn  Numerator=[pi]  Denominator=[30 0]
  Transfer Fcn3 : TransferFcn  Numerator=[pi]  Denominator=[30 0]
  UpperRotor_1_RIGID : Subsystem
  舵偏角° : Scope  NumInputPorts=2
  转速 : Scope  NumInputPorts=2
  F4 : PMIOPort  Side=Left
  wires:
  Transfer Fcn1/1 -> Simulink-PS Converter2/1
  Transfer Fcn3/1 -> Simulink-PS Converter3/1
  Constant8/1 -> Add/2
  Add/1 -> Simulink-PS Converter4/1
  Demux/3 -> Add/1, Radians to Degrees/1  "绿（控制滚转）"
  Constant3/1 -> Add1/2
  Add1/1 -> Simulink-PS Converter5/1
  motors_refout/1 -> Demux/1
  Demux/1 -> 转速/2, Transfer Fcn1/1  "Lower"
  Demux/2 -> 转速/1, Transfer Fcn3/1  "Upper"
  Demux/4 -> Add1/1, Radians to Degrees1/1  "灰（控制俯仰）"
  Radians to Degrees/1 -> 舵偏角°/1  "绿（控制滚转）"
  Radians to Degrees1/1 -> 舵偏角°/2  "灰（控制俯仰）"
  connections:
  Body_1_RIGID/RConn4 -- Revolute/LConn1
  Body_1_RIGID/RConn1 -- Revolute5/LConn1
  LowerRotor_1_RIGID/LConn1 -- Revolute5/RConn1
  Body_1_RIGID/RConn3 -- Revolute1/LConn1
  Revolute/RConn1 -- Rudder1_1_RIGID/LConn1
  Revolute4/RConn1 -- UpperRotor_1_RIGID/LConn1
  Revolute1/RConn1 -- Rudder2_1_RIGID/LConn1
  Body_1_RIGID/RConn2 -- Revolute4/LConn1
  F4/RConn1 -- Body_1_RIGID/LConn1
  Simulink-PS Converter2/RConn1 -- Revolute5/LConn2
  Simulink-PS Converter3/RConn1 -- Revolute4/LConn2
  Simulink-PS Converter4/RConn1 -- Revolute1/LConn2
  Simulink-PS Converter5/RConn1 -- Revolute/LConn2

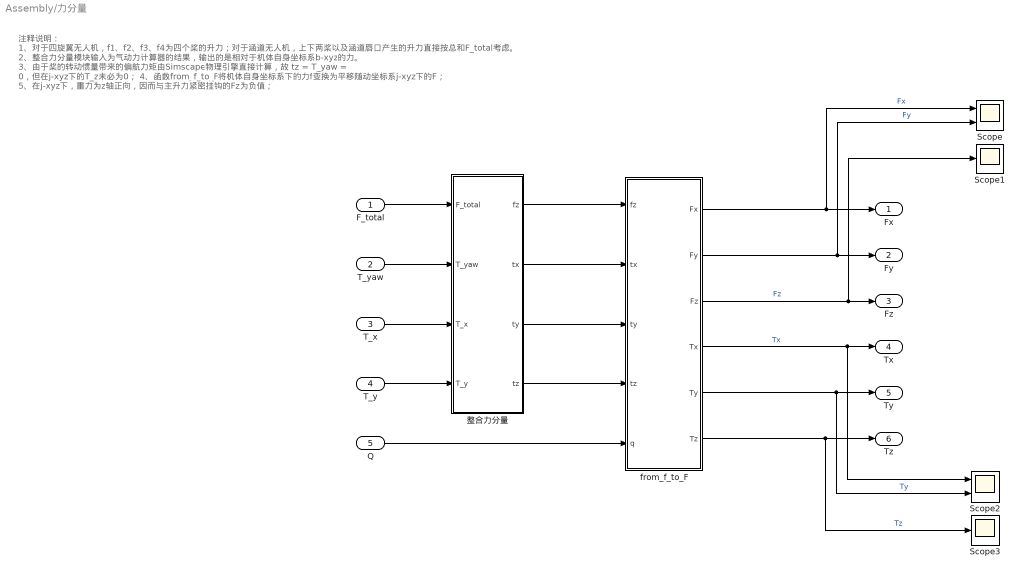
== system Assembly/力分量 ==
  note: 注释说明：
      | 1、对于四旋翼无人机，f1、f2、f3、f4为四个桨的升力；对于涵道无人机，上下两桨以及涵道唇口产生的升力直接按总和F_total考虑。
      | 2、整合力分量模块输入为气动力计算器的结果，输出的是相对于机体自身坐标系b-xyz的力。
      | 3、由于桨的转动惯量带来的偏航力矩由Simscape物理引擎直接计算，故 tz = T_yaw = 0，但在j-xyz下的T_z未必为0；
      | 4、函数from_f_to_F将机体自身坐标系下的力f变换为平移随动坐标系j-xyz下的F；
      | 5、在j-xyz下，重力为z轴正向，因而与主升力紧密挂钩的Fz为负值；
  F_total : Inport
  T_yaw : Inport  Port=2
  T_x : Inport  Port=3
  T_y : Inport  Port=4
  Q : Inport  Port=5
  Scope : Scope  NumInputPorts=2
  Scope1 : Scope
  Scope2 : Scope  NumInputPorts=2
  Scope3 : Scope
  from_f_to_F : MATLAB Function  TreatAsAtomicUnit=on
  整合力分量 : MATLAB Function  TreatAsAtomicUnit=on
  Fx : Outport
  Fy : Outport  Port=2
  Fz : Outport  Port=3
  Tx : Outport  Port=4
  Ty : Outport  Port=5
  Tz : Outport  Port=6
  wires:
  F_total/1 -> 整合力分量/1(F_total)
  T_yaw/1 -> 整合力分量/2(T_yaw)
  T_x/1 -> 整合力分量/3(T_x)
  T_y/1 -> 整合力分量/4(T_y)
  Q/1 -> from_f_to_F/5(q)
  整合力分量/2(tx) -> from_f_to_F/2(tx)
  整合力分量/3(ty) -> from_f_to_F/3(ty)
  from_f_to_F/1(Fx) -> Scope/1, Fx/1  "Fx"
  from_f_to_F/2(Fy) -> Scope/2, Fy/1  "Fy"
  from_f_to_F/3(Fz) -> Scope1/1, Fz/1  "Fz"
  from_f_to_F/4(Tx) -> Scope2/1, Tx/1  "Tx"
  from_f_to_F/5(Ty) -> Scope2/2, Ty/1  "Ty"
  整合力分量/1(fz) -> from_f_to_F/1(fz)
  from_f_to_F/6(Tz) -> Scope3/1, Tz/1  "Tz"
  整合力分量/4(tz) -> from_f_to_F/4(tz)

== system Assembly/升力计算器（注意升力计算结果取正值） ==
  note: 无人机质量4.8239kg
      | 重力47.3225N
  cmd : Inport
  Demux : Demux
  升力 : MATLAB Function  TreatAsAtomicUnit=on
  升力计算 : Subsystem  Commented=on
  舵面力矩 : MATLAB Function  TreatAsAtomicUnit=on
  F_total : Outport
  T_yaw : Outport  Port=2
  T_x : Outport  Port=3
  T_y : Outport  Port=4
  wires:
  升力/1(F_total) -> F_total/1
  升力/2(T_yaw) -> T_yaw/1
  舵面力矩/1(tx) -> T_x/1
  舵面力矩/2(ty) -> T_y/1
  Demux/3 -> 舵面力矩/1(angle_roll)
  Demux/4 -> 舵面力矩/2(angle_pitch)
  cmd/1 -> Demux/1
  Demux/1 -> 升力/1(n1)
  Demux/2 -> 升力/2(n2)

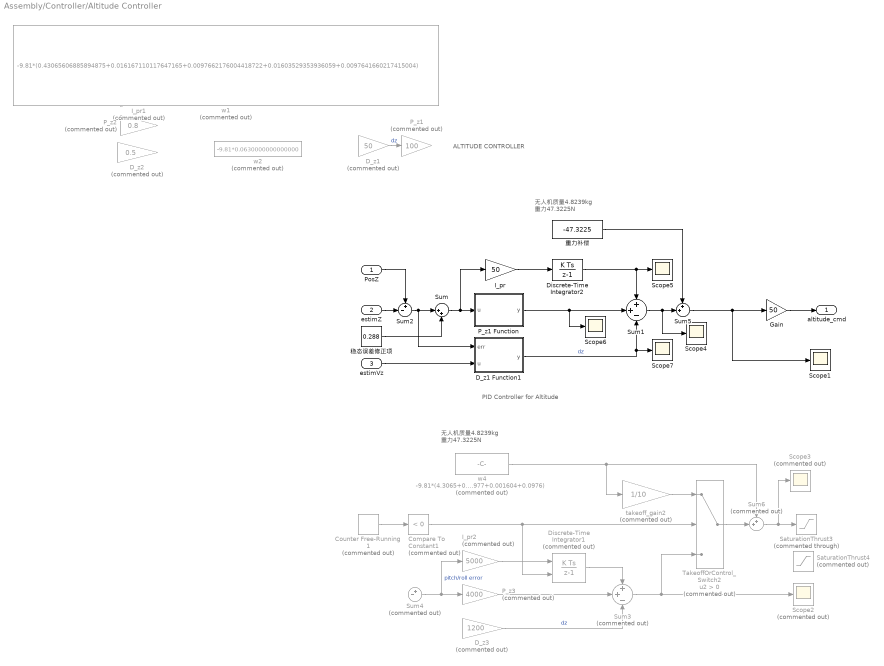
== system Assembly/Controller/Altitude Controller ==
  note: 无人机质量4.8239kg
      | 重力47.3225N
  note: PID Controller for Altitude
  note: ALTITUDE CONTROLLER
  note: 无人机质量4.8239kg
      | 重力47.3225N
  PosZ : Inport
  estimZ : Inport  Port=2
  estimVz : Inport  Port=3
  Compare To Constant1 : simulink/Logic and Bit Operations/Compare To Constant  Commented=on  relop=<  const=0  OutDataTypeStr=boolean
  Counter Free-Running1 : simulink/Sources/Counter Free-Running  Commented=on  NumBits=16  tsamp=-1
  D_z1 : Gain  Commented=on  Gain=50  ParamDataTypeStr=single  OutDataTypeStr=single  SaturateOnIntegerOverflow=on
  D_z1 Function1 : MATLAB Function  TreatAsAtomicUnit=on
  D_z2 : Gain  Commented=on  Gain=0.5  ParamDataTypeStr=single  OutDataTypeStr=single  SaturateOnIntegerOverflow=on
  D_z3 : Gain  Commented=on  Gain=1200  ParamDataTypeStr=single  OutDataTypeStr=single  SaturateOnIntegerOverflow=on
  Discrete-Time Integrator1 : DiscreteIntegrator  Commented=on  ExternalReset=falling  SampleTime=0.005  LimitOutput=on  UpperSaturationLimit=2  LowerSaturationLimit=-2  ICPrevOutput=DiscIntNeverNeededParam  ICPrevScaledInput=DiscIntNeverNeededParam
  Discrete-Time Integrator2 : DiscreteIntegrator  gainval=1  SampleTime=-1  LimitOutput=on  UpperSaturationLimit=2  LowerSaturationLimit=-2  ICPrevOutput=DiscIntNeverNeededParam  ICPrevScaledInput=DiscIntNeverNeededParam
  Gain : Gain  Gain=50
  I_pr : Gain  Gain=50
  I_pr1 : Gain  Commented=on  Gain=0.24
  I_pr2 : Gain  Commented=on  Gain=5000
  P_z1 : Gain  Commented=on  Gain=100  ParamDataTypeStr=single  OutDataTypeStr=single  SaturateOnIntegerOverflow=on
  P_z1 Function : MATLAB Function  TreatAsAtomicUnit=on
  P_z2 : Gain  Commented=on  Gain=0.8  ParamDataTypeStr=single  OutDataTypeStr=single  SaturateOnIntegerOverflow=on
  P_z3 : Gain  Commented=on  Gain=4000  ParamDataTypeStr=single  OutDataTypeStr=single  SaturateOnIntegerOverflow=on
  SaturationThrust3 : Saturate  Commented=through  UpperLimit=10  LowerLimit=-10
  SaturationThrust4 : Saturate  Commented=on  UpperLimit=4*0.920000000000000*0.326642213351703  LowerLimit=-4*0.920000000000000*0.326642213351703
  Scope{1,4..7} (5 alike) : Scope
  Scope2 : Scope  Commented=on
  Scope3 : Scope  Commented=on
  Sum : Sum  Inputs=|++
  Sum1 : Sum  Inputs=++-  AccumDataTypeStr=single  OutDataTypeStr=single  SaturateOnIntegerOverflow=on
  Sum2 : Sum  Inputs=+-|  AccumDataTypeStr=single  OutDataTypeStr=single  SaturateOnIntegerOverflow=on
  Sum3 : Sum  Commented=on  Inputs=++-  AccumDataTypeStr=single  OutDataTypeStr=single  SaturateOnIntegerOverflow=on
  Sum4 : Sum  Commented=on  Inputs=+-|  AccumDataTypeStr=single  OutDataTypeStr=single  SaturateOnIntegerOverflow=on
  Sum5 : Sum  Inputs=++|  AccumDataTypeStr=double  OutDataTypeStr=double  SaturateOnIntegerOverflow=on
  Sum6 : Sum  Commented=on  Inputs=++|  AccumDataTypeStr=double  OutDataTypeStr=double  SaturateOnIntegerOverflow=on
  TakeoffOrControl_Switch2 : Switch  Commented=on  Criteria=u2 > Threshold  SaturateOnIntegerOverflow=off  InputSameDT=off
  takeoff_gain2 : Gain  Commented=on  Gain=1/10  ParamDataTypeStr=single  OutDataTypeStr=double  SaturateOnIntegerOverflow=on
  w1 : Constant  Commented=on  Value=-9.81*(0.43065606885894875+0.016167110117647165+0.0097662176004418722+0.01603529353936059+0.0097641660217415004)  OutDataTypeStr=double  SampleTime=0.005
  w2 : Constant  Commented=on  Value=-9.81*0.0630000000000000  OutDataTypeStr=double  SampleTime=0.005
  w4 : Constant  Commented=on  Value=-9.81*(4.3065+0.001617+0.0977+0.001604+0.0976)  OutDataTypeStr=double  SampleTime=0.005
  稳态误差修正项 : Constant  Value=0.288
  重力补偿 : Constant  Value=-47.3225  OutDataTypeStr=double  SampleTime=0.005
  altitude_cmd : Outport  VectorParamsAs1DForOutWhenUnconnected=off
  wires:
  Discrete-Time Integrator2/1 -> Sum1/1, Scope5/1
  P_z1 Function/1(y) -> Scope6/1, Sum1/2
  D_z1 Function1/1(y) -> Scope7/1, Sum1/3  "dz"
  Sum1/1 -> Scope4/1, Sum5/2
  I_pr/1 -> Discrete-Time Integrator2/1
  重力补偿/1 -> Sum5/1
  Discrete-Time Integrator1/1 -> Sum3/1
  Counter Free-Running1/1 -> Compare To Constant1/1
  w4/1 -> takeoff_gain2/1, Sum6/1
  I_pr2/1 -> Discrete-Time Integrator1/1
  Sum4/1 -> I_pr2/1, P_z3/1  "pitch/roll error"
  Sum6/1 -> Scope3/1, SaturationThrust3/1
  Sum3/1 -> Scope2/1, TakeoffOrControl_Switch2/3
  takeoff_gain2/1 -> TakeoffOrControl_Switch2/1
  Compare To Constant1/1 -> Discrete-Time Integrator1/2, TakeoffOrControl_Switch2/2
  TakeoffOrControl_Switch2/1 -> Sum6/2
  P_z3/1 -> Sum3/2
  D_z3/1 -> Sum3/3  "dz"
  Sum5/1 -> Gain/1, Scope1/1
  PosZ/1 -> Sum2/1
  estimZ/1 -> Sum2/2
  estimVz/1 -> D_z1 Function1/2(u)
  Gain/1 -> altitude_cmd/1
  Sum2/1 -> D_z1 Function1/1(err), Sum/1
  Sum/1 -> I_pr/1, P_z1 Function/1(u)
  稳态误差修正项/1 -> Sum/2
  D_z1/1 -> P_z1/1  "dz"
